simulink model "ecelp_sq"  (Simulink 6.1)
settings: Solver=FixedStepDiscrete  SolverMode=SingleTasking  StartTime=0.0  StopTime=3  RelTol=1e-3
PreLoadFcn:
  | load lpcvocoder.mat;
undefined symbols (not defined in the file): magnitude, poly2lsf
libraries: simulink x26, dspquant2 x26, dspindex x18, dspcelplib x14, dsparch4 x12, dspstat3 x10, dspsrcs4 x9, dspsigops x7, dsplp x5, dspmtrx3 x3, dspbuff3 x2, dspsolvers x1
(part 1 of 4)
settings Model: RequirementInfo=9  CovMetricSettings=d  Creator=The MathWorks Inc.  LastModifiedBy=igor  ExtModeTrigMode=oneshot  ExtModeArmWhenConnect=off  ExtModeAutoUpdateStatusClock=off  ProdHWDeviceType=Specified
settings DataIOCC: LimitDataPoints=off  SaveFormat=Structure  SaveOutput=off  SaveTime=off  SignalLoggingName=sigsOut
settings OptimizationCC: BlockReduction=off  BooleanDataType=off  InlineInvariantSignals=off
settings DebuggingCC: CheckExecutionContextPreStartOutputMsg=on  CheckExecutionContextRuntimeOutputMsg=on  InheritedTsInSrcMsg=none  IntegerOverflowMsg=none
settings HardwareCC: ProdHWDeviceType=Specified

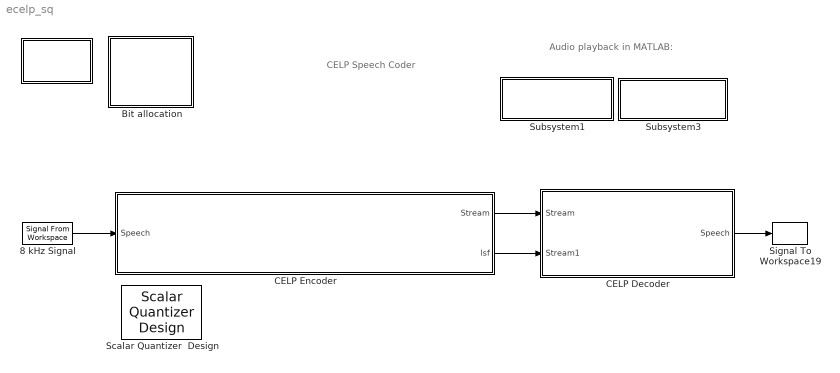
== system ecelp_sq ==
  note: CELP Speech Coder
  note: Audio playback in MATLAB:
  " " : Subsystem
      mask Type: CELP Coder Demo Info
      mask Display: disp('Info')
  "  Bit allocation" : Subsystem  mask(Bit Allocation){bitLSF1to3=10, bitLSF4to6=10, bitLSF7to10=10, bitD=7, bitBeta=6, bitSignGain=4, bitPhase=17, bitAlpha=6}
      mask prompts: bitLSF1to3 "Number of bits for 1st LSF subvector (1 to 3) (per frame):"; bitLSF4to6 "Number of bits for 2nd LSF subvector (4 to 6) (per frame):"; bitLSF7to10 "Number of bits for 3rd LSF subvector (7 to 10) (per frame):"; bitD "Number of bits for Pitch Delay, D (per subframe):"; bitBeta "Number of bits for Pitch Gain, Beta (per subframe):"; bitSignGain "Number of bits for sign of 4 FCB pulses (per subframe):"; bitPhase "Number of bits for position of 4 FCB pulses (per subframe):"; bitAlpha "Number of bits for FCB Gain, Alpha (per subframe):"
      mask help: Bit allocation for the speech coder designed for narrowband speech (sampling frequency 8 KHz) having a frame length of 160 samples and a subframe length of 40 samples (4 subframes per frame).
      mask StyleString: popup(10),popup(10),popup(10),popup(7),popup(6),popup(4),popup(17),popup(6)
      mask Display: disp('Bitrate\n9500 bps')
  8 kHz Signal : dspsrcs4/Signal From Workspace  X=Speech  Ts=1/8000  nsamps=160  OutputAfterFinalValue=Setting to zero
  CELP Decoder : Subsystem
      mask Display:
      | disp('   CELP\n     Decoder')
      | port_label( 'output',1,'Speech' )
      | port_label( 'input', 1, 'dLSFpfc' )
      | port_label( 'input',2,'Other stream' )
  CELP Encoder : Subsystem
      mask Display:
      | disp('CELP\nEncoder')
      | port_label('input',1,'Speech')
      | port_label('output',1,'dequa_LSF per frame content')
      | port_label('output',2,'Other stream')
  Scalar Quantizer  Design : dspquant2/Scalar Quantizer  Design
  Signal To Workspace19 : dspsnks4/Signal To Workspace  VariableName=y_lpc  FrameMode=Concatenate frames (2-D array)
      settings: FixptAsFi=off
  Subsystem1 : Subsystem
      settings: OpenFcn=if exist('Speech','var'), soundsc(Speech,8000); else errordlg('Data not found in workspace - reload demo model.','Signal Processing Blockset Demo Error'); end
      mask Display: disp('Original\nSignal')
  Subsystem3 : Subsystem
      settings: OpenFcn=if exist('y_lpc','var'), soundsc(y_lpc,8000); else uiwait(errordlg('You must run the simulation first.','Signal Processing Blockset Demo Error','modal')); end
      mask Display: disp('Processed\nSignal')
  wires:
  8 kHz Signal/1 -> CELP Encoder/1(Speech)
  CELP Decoder/1(Speech) -> Signal To Workspace19/1
  CELP Encoder/1(Stream) -> CELP Decoder/1(Stream)
  CELP Encoder/2(lsf) -> CELP Decoder/2(Stream1)

== system ecelp_sq/  ==
  note: Code Excited Linear Prediction (CELP) speech coder demo
      |
      | This demo contains a CELP coder composed of an encoder and a decoder.
      |
      | In the encoder, we estimate the parameters of the short-term synthesis
      | filter, the long-term pitch filter and the innovation signal.
      |
      | Using the linear prediction (LP) analysis followed by the quantization and
      | the interpolation of the LSF parameters we calculate the synthesis filter
      | coefficients for each subframe.
      |
      | By applying open loop pitch analysis on the LPC residual signal in each
      | subframe we estimate the pitch predictor delay and the pitch gain
      | parameters.
      |
      | By applying a search on the pitch predictor residual we specify the
      | location and the signs of the FCB (Fixed Code Book) pulses and the FCB
      | gain.
      |
      | To illustrate how the LPC and the pitch analyses remove the short-term and
      | long-term redundancies in the speech signal, the LPC and the pitch residual
      | signals are visualized.
      |
      | The decoder re-synthesizes the speech signal based on the CELP coder
      | parameters contained in the data stream.
      |
      | In this simulation, the speech signal is divided into frames of size 20 ms
      | (160 samples) and each frame is subdivided into four subframes of 5 ms (40
      | samples) each. The bit allocation for each parameter of the coder can be
      | found by double clicking on the 'Bit Allocation' block.
      |
      | The speech phrase used in this demo is from the Harvard list of
      | phonetically balanced sentences, list 14, phrase 8:
      | "Clothes and lodging are free to new men."

== system ecelp_sq/  Bit allocation ==

== system ecelp_sq/CELP Decoder ==
  Stream : Inport  Port=1  LatchInput=off
  Stream1 : Inport  Port=2  LatchInput=off
  Concatenation of subframes to form frame : simulink/Math Operations/Reshape  OutputDimensionality=Customize  OutputDimensions=[160,1]
  Decoding of Data-Stream : dspindex/Multiport Selector  rowsOrCols=Columns  idxCellArray={ 4-3:7-3,8-3:11-3,12-3:27-3,28-3:43-3,44-3:47-3 }  idxErrMode=Clip Index
  Frame to subframe : simulink/Math Operations/Reshape  OutputDimensionality=Customize  OutputDimensions=[4,4]
  LSF Interpolation : Subsystem
  LSF dequantization : Subsystem
  Reshape2 : simulink/Math Operations/Reshape  OutputDimensionality=Customize  OutputDimensions=[4,4]
  Subframe Synthesis : Subsystem  TreatAsAtomicUnit=on
  Speech : Outport
  wires:
  LSF Interpolation/1(LSFinterp) -> Subframe Synthesis/1(lSF_4CH)
  Subframe Synthesis/1(Sigout) -> Concatenation of subframes to form frame/1
  LSF dequantization/1(LSF) -> LSF Interpolation/1(LSF)
  Decoding of Data-Stream/3 -> Frame to subframe/1
  Decoding of Data-Stream/4 -> Reshape2/1
  Decoding of Data-Stream/5 -> Subframe Synthesis/6(Idx_FCBgain)
  Frame to subframe/1 -> Subframe Synthesis/4(4Position)
  Reshape2/1 -> Subframe Synthesis/5(4SignBit)
  Stream/1 -> Decoding of Data-Stream/1
  Concatenation of subframes to form frame/1 -> Speech/1
  Stream1/1 -> LSF dequantization/1(Idx_lsf1to3)
  Decoding of Data-Stream/1 -> Subframe Synthesis/2(Idx_D)
  Decoding of Data-Stream/2 -> Subframe Synthesis/3(Idx_beta)

== system ecelp_sq/CELP Encoder ==
  Speech : Inport  Port=1  LatchInput=off
  DC bias removal : dsparch4/Digital Filter  DialogController=dspDDGCreate  DialogControllerArgs=DataTag12  TypePopup=IIR (poles & zeros)  IIRFiltStruct=Direct form II transposed  AllPoleFiltStruct=Direct form  FIRFiltStruct=Direct form  CoeffSource=Specify via dialog  NumCoeffs="[ 0.9201   -1.8401    0.9201]"  DenCoeffs="[ 1.0000   -1.8337    0.8465]"  BiQuadCoeffs=[1 0.3 0.4 1 0.1 0.2]  LatticeCoeffs=[0.2 0.4]  denIgnore=on  FiltPerSampPopup=One filter per frame  IC=0  ICnum=0  ICden=0  roundingMode=Floor  overflowMode=off  ScaleValues=1  scaleValueFracLength=14  stageInFracLength=15  stageOutFracLength=15
  Data-Stream generation : simulink/Math Operations/Matrix Concatenation  numInports=5  catMethod=Horizontal
  Frame Analysis : Subsystem
  Subframe Analysis : Subsystem  TreatAsAtomicUnit=on
  Stream : Outport
  lsf : Outport  Port=2
  wires:
  Frame Analysis/2(LSF) -> Subframe Analysis/1(LSF)
  DC bias removal/1 -> Frame Analysis/1(FilteredSp), Subframe Analysis/2(Speech)
  Subframe Analysis/5(Idx_FCBgain) -> Data-Stream generation/5
  Data-Stream generation/1 -> Stream/1
  Speech/1 -> DC bias removal/1
  Subframe Analysis/1(Idx_D) -> Data-Stream generation/1
  Subframe Analysis/2(Idx_Beta) -> Data-Stream generation/2
  Subframe Analysis/3(4Position) -> Data-Stream generation/3
  Subframe Analysis/4(4SignBit) -> Data-Stream generation/4
  Frame Analysis/1(IdxLSF) -> lsf/1

== system ecelp_sq/Subsystem1 ==

== system ecelp_sq/Subsystem3 ==

== system ecelp_sq/CELP Decoder/LSF Interpolation ==
  note: LSF Interpolation
  LSF : Inport  Port=1  LatchInput=off
  Delay : dspsigops/Delay  Orientation=down  dly_unit=Frames  delay=1  ic_detail=on  dif_ic_for_ch=off  dif_ic_for_dly=on  ic=(poly2lsf([1 zeros(1,10)])).'  reset_popup=None
  Frame Status : FrameConversion
  Frame Status1 : FrameConversion  OutFrame=Sample based
  Gain : Gain  Orientation=down  Gain=1/4  SaturateOnIntegerOverflow=on
  Matrix Concatenation : simulink/Math Operations/Matrix Concatenation  numInports=4  catMethod=Horizontal
  Sum : Sum  Orientation=down  Inputs=|+-  SaturateOnIntegerOverflow=on
  Sum1 : Sum  Orientation=down  Inputs=++|  SaturateOnIntegerOverflow=on
  Sum2 : Sum  Orientation=down  Inputs=++|  SaturateOnIntegerOverflow=on
  Sum3 : Sum  Inputs=++|  SaturateOnIntegerOverflow=on
  LSFinterp : Outport
  wires:
  LSF/1 -> Frame Status/1
  Sum/1 -> Gain/1
  Sum1/1 -> Matrix Concatenation/1, Sum2/2
  Matrix Concatenation/1 -> Frame Status1/1
  Sum2/1 -> Sum3/1, Matrix Concatenation/2
  Sum3/1 -> Matrix Concatenation/3
  Delay/1 -> Sum1/2, Sum/2
  Gain/1 -> Sum1/1, Sum2/1, Sum3/2
  Frame Status/1 -> Sum/1, Delay/1, Matrix Concatenation/4
  Frame Status1/1 -> LSFinterp/1

== system ecelp_sq/CELP Decoder/LSF dequantization ==
  note: Decoding of LSF sub-vectors
  Idx_lsf1to3 : Inport  Port=1  LatchInput=off
  Sort : dspstat3/Sort  DialogController=dspDDGCreate  DialogControllerArgs=DataTag0  otype=Value  dir=Ascending  sortAlg=Quick sort  roundingMode=Floor  overflowMode=off
  LSF : Outport
  wires:
  Idx_lsf1to3/1 -> Sort/1
  Sort/1 -> LSF/1

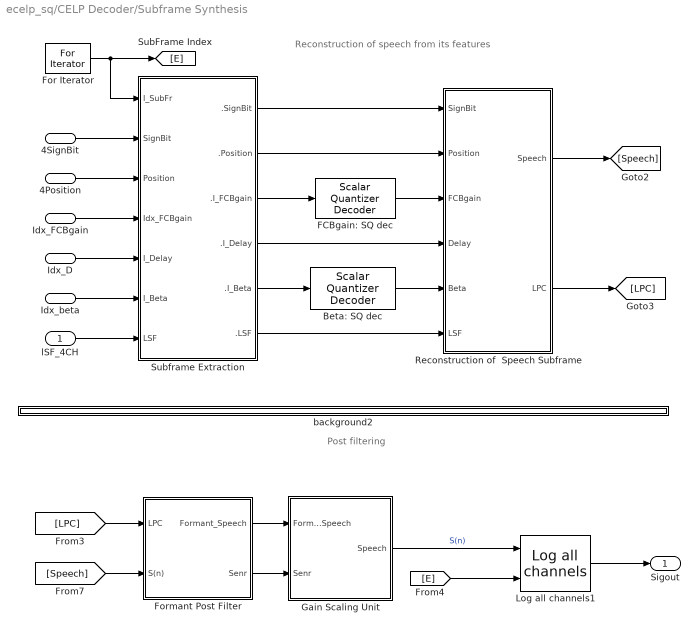
== system ecelp_sq/CELP Decoder/Subframe Synthesis ==
  note: Post filtering
  note: Reconstruction of speech from its features
  lSF_4CH : Inport  Port=1  LatchInput=off
  Idx_D : Inport  Port=2  LatchInput=off
  Idx_beta : Inport  Port=3  LatchInput=off
  4Position : Inport  Port=4  LatchInput=off
  4SignBit : Inport  Port=5  LatchInput=off
  Idx_FCBgain : Inport  Port=6  LatchInput=off
  Beta: SQ dec : dspquant2/Scalar Quantizer Decoder  CBsource=Specify via dialog  invalidin=Clip  codebook="[-1082.3569     -246.64044     -206.60177     -119.68735     -118.12987     -109.71395     -107.74187     -101.39102     -96.836918     -91.269156     -86.372177     -83.198634     -82.501047     -77.265358     -76.499561     -74.506154     -73.162943     -72.064354     -69.588398     -67.441995     -64.571558     -63.949501     -62.716478     -61.876738     -61.311021     -60.518343     -58.650854     -57.975792     -56.936942     -56.282238     -55.386427     -54.862852     -53.494072      -52.94422     -52.032961      -50.72662     -48.968103      -46.10807       -42.6265     -39.065568     -34.843913     -30.198965     -25.969732     -21.578415     -17.256677     -13.047571     -8.5748944     -4.8378646     -2.2872972    -0.86065481    -0.37978458     0.45579633     0.94262874      4.3421606      12.379451      23.629803       37.40066      54.817595      74.624825      93.641473      110.49643      136.97269      179.36351      233.98073]"  dataType=double  isSigned=on  wordLen=16  udDataType=sfix(16)  fracBitsMode=Best precision  numFracBits=11
  FCBgain: SQ dec : dspquant2/Scalar Quantizer Decoder  CBsource=Specify via dialog  invalidin=Clip  codebook="[-0.056021   -0.044097   -0.036312   -0.032845   -0.027656   -0.024334   -0.021157   -0.016236   -0.012644   -0.009939  -0.0075682   -0.005381    -0.00346  -0.0018555 -0.00067033  0.00028187   0.0011099   0.0020196   0.0029919   0.0040377   0.0051592   0.0063683   0.0076408   0.0090117    0.010466    0.012026     0.01376    0.015654    0.017725     0.01998    0.022452    0.025171    0.028043    0.031282    0.034713    0.038275    0.042246    0.046745    0.051613     0.05696     0.06287    0.069146    0.075778    0.082252     0.08972    0.096123     0.10068     0.10407     0.10799     0.11193     0.11573     0.11868     0.12213     0.12664     0.13004     0.13378     0.13772      0.1425     0.14445     0.14843     0.16231     0.16577      0.1698     0.18011]"  dataType=double  isSigned=on  wordLen=16  udDataType=sfix(16)  fracBitsMode=Best precision  numFracBits=11
  For Iterator : ForIterator  IterationLimit=4
  Formant Post Filter : Subsystem
  Gain Scaling Unit : Subsystem
  Log all channels1 : dspcelplib/Log all channels  outType=Matrix  numRow=40  numCol=4  dType=double
  Reconstruction of  Speech Subframe : Subsystem
  Subframe Extraction : Subsystem
  background2 : Subsystem
      mask Display: disp('')
  Sigout : Outport
  wires:
  For Iterator/1 -> [E], Subframe Extraction/1(I_SubFr)
  Subframe Extraction/6(.LSF) -> Reconstruction of  Speech Subframe/6(LSF)
  lSF_4CH/1 -> Subframe Extraction/7(LSF)
  Reconstruction of  Speech Subframe/1(Speech) -> [Speech]
  Idx_beta/1 -> Subframe Extraction/6(I_Beta)
  Subframe Extraction/5(.I_Beta) -> Beta: SQ dec/1
  Idx_D/1 -> Subframe Extraction/5(I_Delay)
  [Speech] -> Formant Post Filter/2(S(n))
  Formant Post Filter/2(Senr) -> Gain Scaling Unit/2(Senr)
  Formant Post Filter/1(Formant_Speech) -> Gain Scaling Unit/1(Formant_Speech)
  [LPC] -> Formant Post Filter/1(LPC)
  Gain Scaling Unit/1(Speech) -> Log all channels1/1  "S(n)"
  Log all channels1/1 -> Sigout/1
  [E] -> Log all channels1/2
  Subframe Extraction/2(.Position) -> Reconstruction of  Speech Subframe/2(Position)
  Subframe Extraction/1(.SignBit) -> Reconstruction of  Speech Subframe/1(SignBit)
  4Position/1 -> Subframe Extraction/3(Position)
  4SignBit/1 -> Subframe Extraction/2(SignBit)
  Idx_FCBgain/1 -> Subframe Extraction/4(Idx_FCBgain)
  Subframe Extraction/3(.I_FCBgain) -> FCBgain: SQ dec/1
  Reconstruction of  Speech Subframe/2(LPC) -> [LPC]
  FCBgain: SQ dec/1 -> Reconstruction of  Speech Subframe/3(FCBgain)
  Subframe Extraction/4(.I_Delay) -> Reconstruction of  Speech Subframe/4(Delay)
  Beta: SQ dec/1 -> Reconstruction of  Speech Subframe/5(Beta)

== system ecelp_sq/CELP Encoder/Frame Analysis ==
  FilteredSp : Inport  Port=1  LatchInput=off
  " " : Subsystem
      mask Type: CELP Coder Demo Info
      mask Display: disp('Info')
  Classical LPC analysis : Subsystem
      mask Display:
      | disp('LPC\nAnalysis');
      | port_label('input',1,'speech');
      | port_label('output',1,'LPC');
  LSF Interpolation : Subsystem
  LSF Vector Quantization : Subsystem
  IdxLSF : Outport
  LSF : Outport  Port=2
  wires:
  Classical LPC analysis/1(LPC) -> LSF Vector Quantization/1(LPC)
  LSF Vector Quantization/1(qLSF) -> LSF Interpolation/1(LSF)
  FilteredSp/1 -> Classical LPC analysis/1(Speech)
  LSF Interpolation/1(LSFinterp) -> LSF/1
  LSF Vector Quantization/2(IdxLSF) -> IdxLSF/1

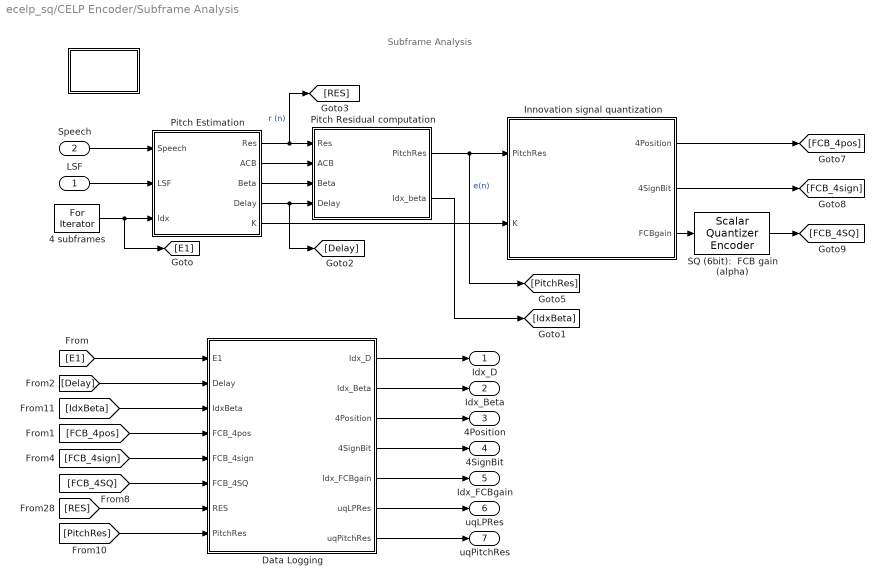
== system ecelp_sq/CELP Encoder/Subframe Analysis ==
  note: Subframe Analysis
  LSF : Inport  Port=1  LatchInput=off
  Speech : Inport  Port=2  LatchInput=off
  " " : Subsystem
      mask Type: CELP Coder Demo Info
      mask Display: disp('Info')
  4 subframes : ForIterator  IterationLimit=4
  Data Logging : Subsystem
  Innovation signal quantization : Subsystem
      mask Display:
      | disp('Pitch\nResidual\nQuantizer');
      | port_label('input',1,'PitchRes');
      | port_label('input',2,'K');
      | port_label('output',1,'4Position');
      | port_label('output',2,'4SignBit');
      | port_label('output',3,'FCBgain');
  Pitch Estimation : Subsystem
  Pitch Residual computation : Subsystem
  SQ (6bit):  FCB gain (alpha) : dspquant2/Scalar Quantizer Encoder  paramSrc=Specify via dialog  partType=Unbounded  BBoundary=[1:10]  UBoundary="[-0.050059   -0.040204   -0.034578   -0.030251   -0.025995   -0.022746   -0.018697    -0.01444   -0.011291  -0.0087536  -0.0064746  -0.0044205  -0.0026578  -0.0012629 -0.00019423  0.00069587   0.0015648   0.0025058   0.0035148   0.0045985   0.0057637   0.0070046   0.0083263   0.0097388    0.011246    0.012893    0.014707    0.016689    0.018853    0.021216    0.023812    0.026607    0.029663    0.032998    0.036494    0.040261    0.044496    0.049179    0.054286    0.059915    0.066008    0.072462    0.079015    0.085986    0.092922    0.098403     0.10238     0.10603     0.10996     0.11383      0.1172     0.12041     0.12439     0.12834     0.13191     0.13575     0.14011     0.14347     0.14644     0.15537     0.16404     0.16779     0.17495]"  SearchMethod=Binary  tieBreakRule=Choose the lower index  outQU=off  outQError=off  codebook="[-1082.3569     -246.64044     -206.60177     -119.68735     -118.12987     -109.71395     -107.74187     -101.39102     -96.836918     -91.269156     -86.372177     -83.198634     -82.501047     -77.265358     -76.499561     -74.506154     -73.162943     -72.064354     -69.588398     -67.441995     -64.571558     -63.949501     -62.716478     -61.876738     -61.311021     -60.518343     -58.650854     -57.975792     -56.936942     -56.282238     -55.386427     -54.862852     -53.494072      -52.94422     -52.032961      -50.72662     -48.968103      -46.10807       -42.6265     -39.065568     -34.843913     -30.198965     -25.969732     -21.578415     -17.256677     -13.047571     -8.5748944     -4.8378646     -2.2872972    -0.86065481    -0.37978458     0.45579633     0.94262874      4.3421606      12.379451      23.629803       37.40066      54.817595      74.624825      93.641473      110.49643      136.97269      179.36351      233.98073]"  outStatus=off  invalidin=Clip  idtype=int32  roundingMode=Floor  overflowMode=off
  Idx_D : Outport
  Idx_Beta : Outport  Port=2
  4Position : Outport  Port=3
  4SignBit : Outport  Port=4
  Idx_FCBgain : Outport  Port=5
  uqLPRes : Outport  Port=6
  uqPitchRes : Outport  Port=7
  wires:
  4 subframes/1 -> [E1], Pitch Estimation/3(Idx)
  Speech/1 -> Pitch Estimation/1(Speech)
  LSF/1 -> Pitch Estimation/2(LSF)
  Data Logging/1(Idx_D) -> Idx_D/1
  [Delay] -> Data Logging/2(Delay)
  Pitch Residual computation/1(PitchRes) -> [PitchRes], Innovation signal quantization/1(PitchRes)  "e(n)"
  Data Logging/2(Idx_Beta) -> Idx_Beta/1
  Data Logging/6(uqLPRes) -> uqLPRes/1
  Data Logging/7(uqPitchRes) -> uqPitchRes/1
  [PitchRes] -> Data Logging/8(PitchRes)
  [RES] -> Data Logging/7(RES)
  Pitch Estimation/5(K) -> Innovation signal quantization/2(K)
  Innovation signal quantization/3(FCBgain) -> SQ (6bit):  FCB gain (alpha)/1
  Data Logging/5(Idx_FCBgain) -> Idx_FCBgain/1
  Data Logging/3(4Position) -> 4Position/1
  Data Logging/4(4SignBit) -> 4SignBit/1
  Pitch Estimation/1(Res) -> Pitch Residual computation/1(Res), [RES]  "r (n)"
  Pitch Estimation/2(ACB) -> Pitch Residual computation/2(ACB)
  Pitch Estimation/3(Beta) -> Pitch Residual computation/3(Beta)
  Pitch Estimation/4(Delay) -> Pitch Residual computation/4(Delay), [Delay]
  Innovation signal quantization/1(4Position) -> [FCB_4pos]
  [FCB_4pos] -> Data Logging/4(FCB_4pos)
  Innovation signal quantization/2(4SignBit) -> [FCB_4sign]
  [FCB_4sign] -> Data Logging/5(FCB_4sign)
  SQ (6bit):  FCB gain (alpha)/1 -> [FCB_4SQ]
  [FCB_4SQ] -> Data Logging/6(FCB_4SQ)
  Pitch Residual computation/2(Idx_beta) -> [IdxBeta]
  [IdxBeta] -> Data Logging/3(IdxBeta)
  [E1] -> Data Logging/1(E1)

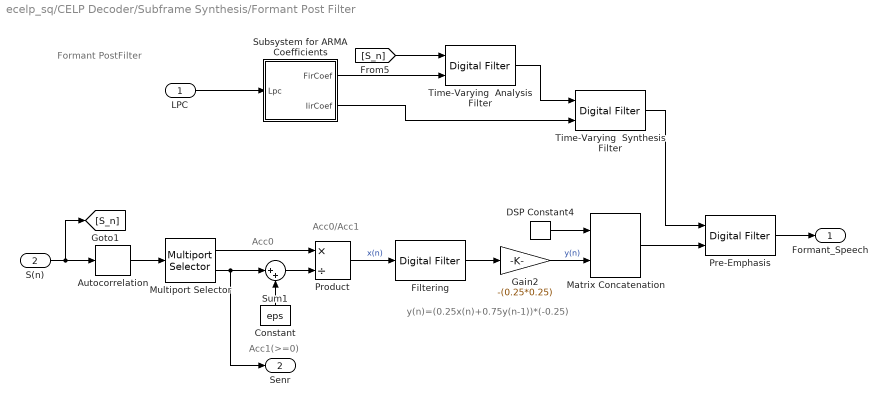
== system ecelp_sq/CELP Decoder/Subframe Synthesis/Formant Post Filter ==
  note: Formant PostFilter
  note: Acc0/Acc1
  note: Acc0
  note: Acc1(>=0)
  note: y(n)=(0.25x(n)+0.75y(n-1))*(-0.25)
  LPC : Inport  Port=1  LatchInput=off
  S(n) : Inport  Port=2  LatchInput=off
  Autocorrelation : dspstat3/Autocorrelation  DialogController=dspDDGCreate  DialogControllerArgs=DataTag1  AllPositiveLags=off  maxlag=1  bias=None  domain=Time  roundingMode=Floor  overflowMode=off
  Constant : Constant  Orientation=up  Value=eps
  DSP Constant4 : dspsrcs4/DSP Constant  Value=1  SampleMode=Discrete  discreteOutput=Sample-based  continuousOutput=Sample-based  sampTime=-1  framePeriod=-1  dataType=double  isSigned=on  wordLen=16  udDataType=sfix(16)  fracBitsMode=Best precision  numFracBits=15  InterpretAs1D=-inf  Ts=-inf  FramebasedOutput=-inf
      settings: additionalParams=on
  Filtering : dsparch4/Digital Filter  DialogController=dspDDGCreate  DialogControllerArgs=DataTag2  TypePopup=IIR (all poles)  IIRFiltStruct=Direct form II transposed  AllPoleFiltStruct=Direct form  FIRFiltStruct=Direct form  CoeffSource=Specify via dialog  NumCoeffs=[1 -.95]  DenCoeffs=[1 -0.75]  BiQuadCoeffs=[1 0.3 0.4 1 0.1 0.2]  LatticeCoeffs=[0.2 0.4]  denIgnore=on  FiltPerSampPopup=One filter per frame  IC=0  ICnum=0  ICden=0  roundingMode=Floor  overflowMode=off  ScaleValues=1  scaleValueFracLength=14  stageInFracLength=15  stageOutFracLength=15
  Gain2 : Gain  Gain=-(0.25*0.25)  SaturateOnIntegerOverflow=on
  Matrix Concatenation : simulink/Math Operations/Matrix Concatenation  numInports=2  catMethod=Vertical
  Multiport Selector : dspindex/Multiport Selector  rowsOrCols=Rows  idxCellArray={2,1}  idxErrMode=Clip Index
  Pre-Emphasis : dsparch4/Digital Filter  DialogController=dspDDGCreate  DialogControllerArgs=DataTag3  TypePopup=FIR (all zeros)  IIRFiltStruct=Direct form II transposed  AllPoleFiltStruct=Direct form  FIRFiltStruct=Direct form  CoeffSource=Input port(s)  NumCoeffs=[1 -.95]  DenCoeffs=[1 0.1]  BiQuadCoeffs=[1 0.3 0.4 1 0.1 0.2]  LatticeCoeffs=[0.2 0.4]  denIgnore=on  FiltPerSampPopup=One filter per frame  IC=0  ICnum=0  ICden=0  roundingMode=Floor  overflowMode=off  ScaleValues=1  scaleValueFracLength=14  stageInFracLength=15  stageOutFracLength=15
  Product : Product  Inputs=*/  SaturateOnIntegerOverflow=on  RndMeth=Zero  InputSameDT=on
  Subsystem for ARMA Coefficients : Subsystem
  Sum1 : Sum  Inputs=|++  SaturateOnIntegerOverflow=on  InputSameDT=on
  Time-Varying  Analysis Filter : dsparch4/Digital Filter  DialogController=dspDDGCreate  DialogControllerArgs=DataTag6  TypePopup=FIR (all zeros)  IIRFiltStruct=Direct form II transposed  AllPoleFiltStruct=Direct form  FIRFiltStruct=Direct form  CoeffSource=Input port(s)  NumCoeffs=[1 -.95]  DenCoeffs=[1 0.1]  BiQuadCoeffs=[1 0.3 0.4 1 0.1 0.2]  LatticeCoeffs=[0.2 0.4]  denIgnore=on  FiltPerSampPopup=One filter per frame  IC=0  ICnum=0  ICden=0  roundingMode=Floor  overflowMode=off  ScaleValues=1  scaleValueFracLength=14  stageInFracLength=15  stageOutFracLength=15
  Time-Varying  Synthesis Filter : dsparch4/Digital Filter  DialogController=dspDDGCreate  DialogControllerArgs=DataTag7  TypePopup=IIR (all poles)  IIRFiltStruct=Direct form II transposed  AllPoleFiltStruct=Direct form  FIRFiltStruct=Direct form  CoeffSource=Input port(s)  NumCoeffs=[1 -.95]  DenCoeffs=[1 0.1]  BiQuadCoeffs=[1 0.3 0.4 1 0.1 0.2]  LatticeCoeffs=[0.2 0.4]  denIgnore=on  FiltPerSampPopup=One filter per frame  IC=0  ICnum=0  ICden=0  roundingMode=Floor  overflowMode=off  ScaleValues=1  scaleValueFracLength=14  stageInFracLength=15  stageOutFracLength=15
  Formant_Speech : Outport
  Senr : Outport  Port=2
  wires:
  LPC/1 -> Subsystem for ARMA Coefficients/1(Lpc)
  Autocorrelation/1 -> Multiport Selector/1
  S(n)/1 -> Autocorrelation/1, [S_n]
  Subsystem for ARMA Coefficients/2(IirCoef) -> Time-Varying  Synthesis Filter/2
  Subsystem for ARMA Coefficients/1(FirCoef) -> Time-Varying  Analysis Filter/2
  Multiport Selector/2 -> Sum1/1, Senr/1
  Multiport Selector/1 -> Product/1
  Time-Varying  Analysis Filter/1 -> Time-Varying  Synthesis Filter/1
  [S_n] -> Time-Varying  Analysis Filter/1
  Time-Varying  Synthesis Filter/1 -> Pre-Emphasis/1
  Matrix Concatenation/1 -> Pre-Emphasis/2
  DSP Constant4/1 -> Matrix Concatenation/1
  Gain2/1 -> Matrix Concatenation/2  "y(n)"
  Pre-Emphasis/1 -> Formant_Speech/1
  Sum1/1 -> Product/2
  Constant/1 -> Sum1/2
  Product/1 -> Filtering/1  "x(n)"
  Filtering/1 -> Gain2/1

== system ecelp_sq/CELP Decoder/Subframe Synthesis/Gain Scaling Unit ==
  note: Gain Scaling Unit
  note: Senr
  note: Acc1
  Formant_Speech : Inport  Port=1  LatchInput=off
  Senr : Inport  Port=2  LatchInput=off
  0.0625 : dspsrcs4/DSP Constant  Value=1/16  SampleMode=Discrete  discreteOutput=Sample-based  continuousOutput=Sample-based  sampTime=-1  framePeriod=-1  dataType=Inherit from 'Constant value'  isSigned=on  wordLen=16  udDataType=sfix(16)  fracBitsMode=Best precision  numFracBits=15  InterpretAs1D=off  Ts=-1  FramebasedOutput=off
  1.0625 : Constant  Value=17/16
  Dot Product : simulink/Math Operations/Dot Product  OutDataType=sfix(16)  OutScaling=2^-10  DoSatur=on
  For Iterator Subsystem1 : Subsystem  TreatAsAtomicUnit=on
  Gain2 : Gain  Gain=1/16  SaturateOnIntegerOverflow=on
  Product : Product  Inputs=*/  SaturateOnIntegerOverflow=on  RndMeth=Zero  InputSameDT=on
  Product1 : Product  Inputs=3  SaturateOnIntegerOverflow=on  RndMeth=Zero  InputSameDT=on
  Switch1 : Switch  Threshold=1.175494351e-38  SaturateOnIntegerOverflow=on  InputSameDT=on
  sqrt(Senr/Acc1) : Math  Operator=sqrt  SaturateOnIntegerOverflow=on
  Speech : Outport
  wires:
  Senr/1 -> Product/1
  Switch1/1 -> For Iterator Subsystem1/1(ScalarGain)
  Gain2/1 -> Switch1/1
  0.0625/1 -> Switch1/3
  sqrt(Senr/Acc1)/1 -> Gain2/1
  Product/1 -> sqrt(Senr/Acc1)/1
  Dot Product/1 -> Switch1/2, Product/2
  Formant_Speech/1 -> Dot Product/1, Dot Product/2, Product1/2
  1.0625/1 -> Product1/3
  For Iterator Subsystem1/1(VectorGain) -> Product1/1
  Product1/1 -> Speech/1

== system ecelp_sq/CELP Decoder/Subframe Synthesis/Reconstruction of  Speech Subframe ==
  SignBit : Inport  Port=1  LatchInput=off
  Position : Inport  Port=2  LatchInput=off
  FCBgain : Inport  Port=3  LatchInput=off
  Delay : Inport  Port=4  LatchInput=off
  Beta : Inport  Port=5  LatchInput=off
  LSF : Inport  Port=6  LatchInput=off
  Harmonic Shaper : Subsystem
  LP Synthesis Filter : Subsystem
  Pitch synthesis : Subsystem
  Reconstruction of  Pitch Residual Signal : Subsystem
  Speech : Outport
  LPC : Outport  Port=2
  wires:
  Delay/1 -> Harmonic Shaper/2(Delay), Pitch synthesis/2(Delay)
  Beta/1 -> Harmonic Shaper/3(Beta), Pitch synthesis/3(Beta)
  Harmonic Shaper/1(OutRes) -> LP Synthesis Filter/1(Residual)
  Reconstruction of  Pitch Residual Signal/1(qPitchRes) -> Pitch synthesis/1(PitchRes)
  Pitch synthesis/1(LPRes) -> Harmonic Shaper/1(inRes)
  SignBit/1 -> Reconstruction of  Pitch Residual Signal/1(4SignBit)
  Position/1 -> Reconstruction of  Pitch Residual Signal/2(4Position)
  FCBgain/1 -> Reconstruction of  Pitch Residual Signal/3(FCBgain)
  LP Synthesis Filter/1(Sig) -> Speech/1  "S(n)"
  LSF/1 -> LP Synthesis Filter/2(LSF)
  LP Synthesis Filter/2(LPC) -> LPC/1

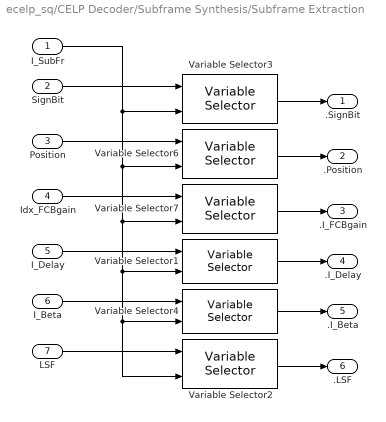
== system ecelp_sq/CELP Decoder/Subframe Synthesis/Subframe Extraction ==
  I_SubFr : Inport  Port=1  LatchInput=off
  SignBit : Inport  Port=2  LatchInput=off
  Position : Inport  Port=3  LatchInput=off
  Idx_FCBgain : Inport  Port=4  LatchInput=off
  I_Delay : Inport  Port=5  LatchInput=off
  I_Beta : Inport  Port=6  LatchInput=off
  LSF : Inport  Port=7  LatchInput=off
  Variable Selector1 : dspindex/Variable Selector  rowsOrCols=Columns  IdxMode=Variable  Elements=[1 3]  ZerOneIdxMode=One-based  errmode=Clip Index
  Variable Selector2 : dspindex/Variable Selector  rowsOrCols=Columns  IdxMode=Variable  Elements=[1 3]  ZerOneIdxMode=One-based  errmode=Clip Index
  Variable Selector3 : dspindex/Variable Selector  rowsOrCols=Columns  IdxMode=Variable  Elements=[1 3]  ZerOneIdxMode=One-based  errmode=Generate Error
  Variable Selector4 : dspindex/Variable Selector  rowsOrCols=Columns  IdxMode=Variable  Elements=[1 3]  ZerOneIdxMode=One-based  errmode=Clip Index
  Variable Selector6 : dspindex/Variable Selector  rowsOrCols=Columns  IdxMode=Variable  Elements=[1 3]  ZerOneIdxMode=One-based  errmode=Generate Error
  Variable Selector7 : dspindex/Variable Selector  rowsOrCols=Columns  IdxMode=Variable  Elements=[1 3]  ZerOneIdxMode=One-based  errmode=Generate Error
  .SignBit : Outport
  .Position : Outport  Port=2
  .I_FCBgain : Outport  Port=3
  .I_Delay : Outport  Port=4
  .I_Beta : Outport  Port=5
  .LSF : Outport  Port=6
  wires:
  I_SubFr/1 -> Variable Selector3/2, Variable Selector6/2, Variable Selector2/2, Variable Selector4/2, Variable Selector1/2, Variable Selector7/2
  SignBit/1 -> Variable Selector3/1
  Variable Selector3/1 -> .SignBit/1
  Position/1 -> Variable Selector6/1
  Variable Selector6/1 -> .Position/1
  Idx_FCBgain/1 -> Variable Selector7/1
  Variable Selector7/1 -> .I_FCBgain/1
  I_Delay/1 -> Variable Selector1/1
  Variable Selector1/1 -> .I_Delay/1
  I_Beta/1 -> Variable Selector4/1
  Variable Selector4/1 -> .I_Beta/1
  LSF/1 -> Variable Selector2/1
  Variable Selector2/1 -> .LSF/1

== system ecelp_sq/CELP Decoder/Subframe Synthesis/background2 ==

== system ecelp_sq/CELP Encoder/Frame Analysis/  ==
  note: Frame analysis is composed of three steps:
      |
      | 1. Classical LPC analysis
      | 2. Split vector quantization of LSF vector
      | 3. LSF interpolation

== system ecelp_sq/CELP Encoder/Frame Analysis/Classical LPC analysis ==
  note: LPC Analysis
  Speech : Inport  Port=1  LatchInput=off
  " " : Subsystem
      mask Type: CELP Coder Demo Info
      mask Display: disp('Info')
  Autocorrelation : dspstat3/Autocorrelation  DialogController=dspDDGCreate  DialogControllerArgs=DataTag13  AllPositiveLags=off  maxlag=10  bias=Biased  domain=Time  roundingMode=Floor  overflowMode=off
  Bandwidth Expansion : Subsystem  mask(Bandwidth Expansion){alpha=0.994}
      mask prompts: alpha "Bandwidth expansion factor:"
      mask help:
      | Generate autoregressive (AR) polynomial with bandwidth expanded relative to the bandwidth of the input AR polynomial.
      |
      | By reducing the radius of the roots in an autoregressive polynomial (i.e., scaling them towards the origin of the Z-plane), the bandwidth of the spectral peaks in the frequency response is expanded (flattened).  This operation is often referred to as "bandwidth expansion".
      |
      | Bandwidth expansion factor must be in the range [0,1], where 1.0 yields no changes to the roots of the polynomial.
      mask Help: web(dspbhelp);
      mask Display: fprintf('Bandwidth\nExpansion\n%g', alpha)
  Levinson- Durbin : dspsolvers/Levinson-Durbin  DialogController=dspDDGCreate  DialogControllerArgs=DataTag15  coeffOutFcn=A  outP=off  zeroInpHandling=on  firstCoeffMode=Binary point scaling  firstCoeffWordLength=16  firstCoeffFracLength=15  secondCoeffMode=Binary point scaling  secondCoeffWordLength=16  secondCoeffFracLength=15  roundingMode=Floor  overflowMode=off
      settings: allowOverrides=off
  Overlap Analysis Windows : dspbuff3/Buffer  N=240  V=80  ic=0
  Window : dspsigops/Window Function  DialogController=dspDDGCreate  DialogControllerArgs=DataTag16  winmode=Apply window to input  wintype=Hamming  sampmode=Continuous  samptime=1  N=64  Rs=50  beta=10  winsamp=Symmetric  UserWindow=hamming  OptParams=off  UserParams={1.0}  dataType=double  isSigned=on  wordLen=16  udDataType=sfix(16)  fracBitsMode=Best precision  numFracBits=15  roundingMode=Floor  overflowMode=off
  LPC : Outport
  wires:
  Overlap Analysis Windows/1 -> Window/1
  Autocorrelation/1 -> Levinson- Durbin/1
  Window/1 -> Autocorrelation/1
  Speech/1 -> Overlap Analysis Windows/1
  Levinson- Durbin/1 -> Bandwidth Expansion/1(In1)
  Bandwidth Expansion/1(Out1) -> LPC/1

== system ecelp_sq/CELP Encoder/Frame Analysis/LSF Interpolation ==
  note: LSF Interpolation
  LSF : Inport  Port=1  LatchInput=off
  " " : Subsystem
      mask Type: CELP Coder Demo Info
      mask Display: disp('Info')
  Delay : dspsigops/Delay  Orientation=down  dly_unit=Frames  delay=1  ic_detail=on  dif_ic_for_ch=off  dif_ic_for_dly=on  ic=(poly2lsf([1 zeros(1,10)])).'  reset_popup=None
  Frame Status : FrameConversion
  Frame Status1 : FrameConversion  OutFrame=Sample based
  Gain : Gain  Orientation=down  Gain=1/4  SaturateOnIntegerOverflow=on
  Matrix Concatenation : simulink/Math Operations/Matrix Concatenation  numInports=4  catMethod=Horizontal
  Sum : Sum  Orientation=down  Inputs=|+-  SaturateOnIntegerOverflow=on
  Sum1 : Sum  Orientation=down  Inputs=++|  SaturateOnIntegerOverflow=on
  Sum2 : Sum  Orientation=down  Inputs=++|  SaturateOnIntegerOverflow=on
  Sum3 : Sum  Inputs=++|  SaturateOnIntegerOverflow=on
  LSFinterp : Outport
  wires:
  Frame Status/1 -> Sum/1, Delay/1, Matrix Concatenation/4
  Sum/1 -> Gain/1
  Sum1/1 -> Matrix Concatenation/1, Sum2/2
  Matrix Concatenation/1 -> Frame Status1/1
  Sum2/1 -> Sum3/1, Matrix Concatenation/2
  Sum3/1 -> Matrix Concatenation/3
  Delay/1 -> Sum1/2, Sum/2
  Gain/1 -> Sum1/1, Sum2/1, Sum3/2
  LSF/1 -> Frame Status/1
  Frame Status1/1 -> LSFinterp/1

== system ecelp_sq/CELP Encoder/Frame Analysis/LSF Vector Quantization ==
  note: Split Vector Quantization of LSF vector
  LPC : Inport  Port=1  LatchInput=off
  " " : Subsystem
      mask Type: CELP Coder Demo Info
      mask Display: disp('Info')
  LPC to LSF  conversion : dsplp/LPC to LSF//LSP Conversion  output=LSF in range (0 pi)  NSteps=64  NBisects=4  RootStatus=off  correction=off  lastLSP=off  error=Ignore
  LSF xQ. : Subsystem
  Paliwal Weight  Computation : Subsystem
  Reshape1 : simulink/Math Operations/Reshape  OutputDimensionality=Column vector  OutputDimensions=[1,1]
  qLSF : Outport
  IdxLSF : Outport  Port=2
  wires:
  LPC/1 -> Reshape1/1
  Paliwal Weight  Computation/1(Weights) -> LSF xQ./2(W1to10)
  Reshape1/1 -> LPC to LSF  conversion/1, Paliwal Weight  Computation/2(LPC)
  LPC to LSF  conversion/1 -> Paliwal Weight  Computation/1(LSF), LSF xQ./1(U1to10)
  LSF xQ./1(qLSF) -> qLSF/1
  LSF xQ./2(IdxLSF) -> IdxLSF/1

== system ecelp_sq/CELP Encoder/Subframe Analysis/  ==
  note: Subframe analysis is composed of three steps:
      |
      | 1. Pitch estimation
      | 2. Pitch residual (innovation signal) computation
      | 3. Innovation signal quantization using fixed codebook

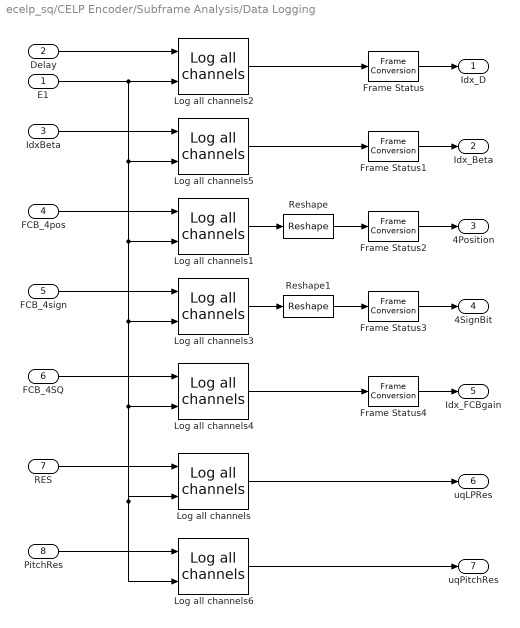
== system ecelp_sq/CELP Encoder/Subframe Analysis/Data Logging ==
  E1 : Inport  Port=1  LatchInput=off
  Delay : Inport  Port=2  LatchInput=off
  IdxBeta : Inport  Port=3  LatchInput=off
  FCB_4pos : Inport  Port=4  LatchInput=off
  FCB_4sign : Inport  Port=5  LatchInput=off
  FCB_4SQ : Inport  Port=6  LatchInput=off
  RES : Inport  Port=7  LatchInput=off
  PitchRes : Inport  Port=8  LatchInput=off
  Frame Status{,1..4} (5 alike) : FrameConversion  OutFrame=Sample based
  Log all channels : dspcelplib/Log all channels  outType=Matrix  numRow=40  numCol=4  dType=double
  Log all channels1 : dspcelplib/Log all channels  outType=Matrix  numRow=4  numCol=4  dType=int32
  Log all channels2 : dspcelplib/Log all channels  outType=Row vector  numRow=40  numCol=4  dType=int32
  Log all channels3 : dspcelplib/Log all channels  outType=Matrix  numRow=4  numCol=4  dType=int32
  Log all channels4 : dspcelplib/Log all channels  outType=Row vector  numRow=40  numCol=4  dType=int32
  Log all channels5 : dspcelplib/Log all channels  outType=Row vector  numRow=40  numCol=4  dType=int32
  Log all channels6 : dspcelplib/Log all channels  outType=Matrix  numRow=40  numCol=4  dType=double
  Reshape : simulink/Math Operations/Reshape  OutputDimensionality=Customize  OutputDimensions=[1,16]
  Reshape1 : simulink/Math Operations/Reshape  OutputDimensionality=Customize  OutputDimensions=[1,16]
  Idx_D : Outport
  Idx_Beta : Outport  Port=2
  4Position : Outport  Port=3
  4SignBit : Outport  Port=4
  Idx_FCBgain : Outport  Port=5
  uqLPRes : Outport  Port=6
  uqPitchRes : Outport  Port=7
  wires:
  E1/1 -> Log all channels/2, Log all channels6/2, Log all channels4/2, Log all channels3/2, Log all channels1/2, Log all channels5/2, Log all channels2/2
  Log all channels1/1 -> Reshape/1
  Log all channels3/1 -> Reshape1/1
  Delay/1 -> Log all channels2/1
  Log all channels2/1 -> Frame Status/1
  IdxBeta/1 -> Log all channels5/1
  Log all channels5/1 -> Frame Status1/1
  FCB_4pos/1 -> Log all channels1/1
  Reshape/1 -> Frame Status2/1
  FCB_4sign/1 -> Log all channels3/1
  Reshape1/1 -> Frame Status3/1
  FCB_4SQ/1 -> Log all channels4/1
  Log all channels4/1 -> Frame Status4/1
  RES/1 -> Log all channels/1
  Log all channels/1 -> uqLPRes/1
  PitchRes/1 -> Log all channels6/1
  Log all channels6/1 -> uqPitchRes/1
  Frame Status/1 -> Idx_D/1
  Frame Status1/1 -> Idx_Beta/1
  Frame Status2/1 -> 4Position/1
  Frame Status3/1 -> 4SignBit/1
  Frame Status4/1 -> Idx_FCBgain/1

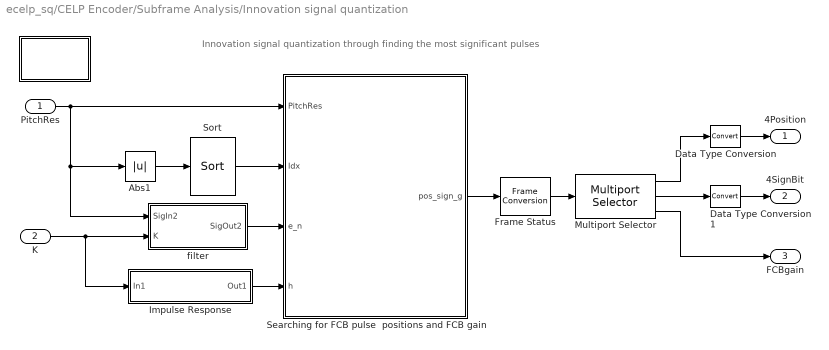
== system ecelp_sq/CELP Encoder/Subframe Analysis/Innovation signal quantization ==
  note: Innovation signal quantization through finding the most significant pulses
  PitchRes : Inport  Port=1  LatchInput=off
  K : Inport  Port=2  LatchInput=off
  " " : Subsystem
      mask Type: CELP Coder Demo Info
      mask Display: disp('Info')
  Abs1 : Abs  SaturateOnIntegerOverflow=on
  Data Type Conversion : DataTypeConversion  OutDataTypeMode=int32  SaturateOnIntegerOverflow=on  RndMeth=Zero
  Data Type Conversion1 : DataTypeConversion  OutDataTypeMode=int32  SaturateOnIntegerOverflow=on  RndMeth=Zero
  Frame Status : FrameConversion  OutFrame=Sample based
  Impulse Response : Subsystem
      mask Display:
      | disp('Impulse Response');
      | port_label('input',1,'K');
      | port_label('output',1,'h');
  Multiport Selector : dspindex/Multiport Selector  rowsOrCols=Rows  idxCellArray={ 1:4,5:8,9 }  idxErrMode=Generate Error
  Searching for FCB pulse  positions and FCB gain : Subsystem  TreatAsAtomicUnit=on
  Sort : dspstat3/Sort  DialogController=dspDDGCreate  DialogControllerArgs=DataTag21  otype=Index  dir=Descending  sortAlg=Quick sort  roundingMode=Floor  overflowMode=off
  filter : Subsystem  TreatAsAtomicUnit=on
      mask Display:
      | disp('Zero State\nIIR Lattice\nFilter');
      | port_label('input',1,'In');
      | port_label('input',2,'K');
      | port_label('output',1,'Out');
  4Position : Outport
  4SignBit : Outport  Port=2
  FCBgain : Outport  Port=3
  wires:
  Impulse Response/1(Out1) -> Searching for FCB pulse  positions and FCB gain/4(h)
  filter/1(SigOut2) -> Searching for FCB pulse  positions and FCB gain/3(e_n)
  K/1 -> Impulse Response/1(In1), filter/2(K)
  Multiport Selector/3 -> FCBgain/1
  Data Type Conversion1/1 -> 4SignBit/1
  Data Type Conversion/1 -> 4Position/1
  Sort/1 -> Searching for FCB pulse  positions and FCB gain/2(Idx)
  Abs1/1 -> Sort/1
  PitchRes/1 -> filter/1(SigIn2), Abs1/1, Searching for FCB pulse  positions and FCB gain/1(PitchRes)
  Multiport Selector/2 -> Data Type Conversion1/1
  Multiport Selector/1 -> Data Type Conversion/1
  Searching for FCB pulse  positions and FCB gain/1(pos_sign_g) -> Frame Status/1
  Frame Status/1 -> Multiport Selector/1

== system ecelp_sq/CELP Encoder/Subframe Analysis/Pitch Estimation ==
  note: Pitch Estimation
  Speech : Inport  Port=1  LatchInput=off
  LSF : Inport  Port=2  LatchInput=off
  Idx : Inport  Port=3  LatchInput=off
  " " : Subsystem
      mask Type: CELP Coder Demo Info
      mask Display: disp('Info')
  Frame Status : FrameConversion  OutFrame=Sample based
  LPC Residual Buffer : dspbuff3/Buffer  N=128+40+20-1  V=187-40  ic=0
  LPC Residual Calculation : Subsystem
  Open loop  Pitch estimation : Subsystem
  Subframe Extraction : Subsystem
  Res : Outport
  ACB : Outport  Port=2
  Beta : Outport  Port=3
  Delay : Outport  Port=4
  K : Outport  Port=5
  wires:
  Subframe Extraction/1(Speech.) -> LPC Residual Calculation/1(Speech)
  Subframe Extraction/2(LSF.) -> LPC Residual Calculation/2(LSF)
  LPC Residual Calculation/1(Residual) -> LPC Residual Buffer/1, Open loop  Pitch estimation/2(Res), Res/1  "r (n)"
  LPC Residual Buffer/1 -> Frame Status/1
  Speech/1 -> Subframe Extraction/1(Speech)
  Open loop  Pitch estimation/1(Beta) -> Beta/1
  LSF/1 -> Subframe Extraction/2(LSF)
  LPC Residual Calculation/2(K) -> K/1
  Idx/1 -> Subframe Extraction/3(SubFrIdx)
  Open loop  Pitch estimation/2(Delay) -> Delay/1
  Frame Status/1 -> ACB/1, Open loop  Pitch estimation/1(ACB)

== system ecelp_sq/CELP Encoder/Subframe Analysis/Pitch Residual computation ==
  note: r (n-D)
  note: beta.r (n-D)
  Res : Inport  Port=1  LatchInput=off
  ACB : Inport  Port=2  LatchInput=off
  Beta : Inport  Port=3  LatchInput=off
  Delay : Inport  Port=4  LatchInput=off
  " " : Subsystem
      mask Type: CELP Coder Demo Info
      mask Display: disp('Info')
  Adaptive codebook (ACB) vector candidate  generation : dspcelplib/Select Rows  numRows=40
  Frame Status : FrameConversion  OutFrame=Sample based
  Product : Product  SaturateOnIntegerOverflow=on  InputSameDT=on
  SQ (6bits):  Pitch gain (beta) : dspquant2/Scalar Quantizer Encoder  paramSrc=Specify via dialog  partType=Unbounded  BBoundary=[1:10]  UBoundary="[-664.4987     -226.6211     -163.1446     -118.9086     -113.9219     -108.7279     -104.5664     -99.11397     -94.05304     -88.82067     -84.78541     -82.84984      -79.8832     -76.88246     -75.50286     -73.83455     -72.61365     -70.82638      -68.5152     -66.00678     -64.26053     -63.33299     -62.29661     -61.59388     -60.91468      -59.5846     -58.31332     -57.45637     -56.60959     -55.83433     -55.12464     -54.17846     -53.21915     -52.48859     -51.37979     -49.84736     -47.53809     -44.36728     -40.84603     -36.95474     -32.52144     -28.08435     -23.77407     -19.41755     -15.15212     -10.81123      -6.70638     -3.562581     -1.573976    -0.6202197    0.03800587     0.6992125      2.642395      8.360806      18.00463      30.51523      46.10913      64.72121      84.13315       102.069      123.7346      158.1681      206.6721]"  SearchMethod=Binary  tieBreakRule=Choose the lower index  outQU=on  outQError=off  codebook="[-1082.3569     -246.64044     -206.60177     -119.68735     -118.12987     -109.71395     -107.74187     -101.39102     -96.836918     -91.269156     -86.372177     -83.198634     -82.501047     -77.265358     -76.499561     -74.506154     -73.162943     -72.064354     -69.588398     -67.441995     -64.571558     -63.949501     -62.716478     -61.876738     -61.311021     -60.518343     -58.650854     -57.975792     -56.936942     -56.282238     -55.386427     -54.862852     -53.494072      -52.94422     -52.032961      -50.72662     -48.968103      -46.10807       -42.6265     -39.065568     -34.843913     -30.198965     -25.969732     -21.578415     -17.256677     -13.047571     -8.5748944     -4.8378646     -2.2872972    -0.86065481    -0.37978458     0.45579633     0.94262874      4.3421606      12.379451      23.629803       37.40066      54.817595      74.624825      93.641473      110.49643      136.97269      179.36351      233.98073]"  outStatus=off  invalidin=Clip  idtype=int32  roundingMode=Floor  overflowMode=off
  Sum2 : Sum  Inputs=|+-  SaturateOnIntegerOverflow=on
  PitchRes : Outport
  Idx_beta : Outport  Port=2
  wires:
  ACB/1 -> Adaptive codebook (ACB) vector candidate  generation/1
  Sum2/1 -> Frame Status/1
  Res/1 -> Sum2/1  "r(n)"
  Delay/1 -> Adaptive codebook (ACB) vector candidate  generation/2
  Product/1 -> Sum2/2
  Adaptive codebook (ACB) vector candidate  generation/1 -> Product/1
  Beta/1 -> SQ (6bits):  Pitch gain (beta)/1
  SQ (6bits):  Pitch gain (beta)/2 -> Product/2
  SQ (6bits):  Pitch gain (beta)/1 -> Idx_beta/1
  Frame Status/1 -> PitchRes/1

== system ecelp_sq/CELP Decoder/Subframe Synthesis/Formant Post Filter/Subsystem for ARMA Coefficients ==
  Lpc : Inport  Port=1  LatchInput=off
  Bandwidth Expansion : Subsystem  mask(Bandwidth Expansion){alpha=0.65}
      mask prompts: alpha "Bandwidth expansion factor:"
      mask help:
      | Generate autoregressive (AR) polynomial with bandwidth expanded relative to the bandwidth of the input AR polynomial.
      |
      | By reducing the radius of the roots in an autoregressive polynomial (i.e., scaling them towards the origin of the Z-plane), the bandwidth of the spectral peaks in the frequency response is expanded (flattened).  This operation is often referred to as "bandwidth expansion".
      |
      | Bandwidth expansion factor must be in the range [0,1], where 1.0 yields no changes to the roots of the polynomial.
      mask Help: web(dspbhelp);
      mask Display: fprintf('Bandwidth\nExpansion\n%g', alpha)
  Bandwidth Expansion1 : Subsystem  mask(Bandwidth Expansion){alpha=0.75}
      mask prompts: alpha "Bandwidth expansion factor:"
      mask help:
      | Generate autoregressive (AR) polynomial with bandwidth expanded relative to the bandwidth of the input AR polynomial.
      |
      | By reducing the radius of the roots in an autoregressive polynomial (i.e., scaling them towards the origin of the Z-plane), the bandwidth of the spectral peaks in the frequency response is expanded (flattened).  This operation is often referred to as "bandwidth expansion".
      |
      | Bandwidth expansion factor must be in the range [0,1], where 1.0 yields no changes to the roots of the polynomial.
      mask Help: web(dspbhelp);
      mask Display: fprintf('Bandwidth\nExpansion\n%g', alpha)
  FirCoef : Outport
  IirCoef : Outport  Port=2
  wires:
  Lpc/1 -> Bandwidth Expansion/1(In1), Bandwidth Expansion1/1(In1)
  Bandwidth Expansion1/1(Out1) -> IirCoef/1
  Bandwidth Expansion/1(Out1) -> FirCoef/1

== system ecelp_sq/CELP Decoder/Subframe Synthesis/Gain Scaling Unit/For Iterator Subsystem1 ==
  note: g(n)
  note: y(n)
  note: y(n)=g(n)+0.9375y(n-1)
      | with IC=1
  note: Computation of gain scaling factor for each sample of the subframe
  ScalarGain : Inport  Port=1  LatchInput=off
  Assignment : Assignment  ElementSrc=External  Rows=-1  ColumnSrc=External
  Constant1 : Constant  Orientation=down  Value=zeros(40,1)  VectorParams1D=off
  For Iterator : ForIterator  IterationLimit=40
  filter : dsparch4/Digital Filter  DialogController=dspDDGCreate  DialogControllerArgs=DataTag8  TypePopup=IIR (all poles)  IIRFiltStruct=Direct form II transposed  AllPoleFiltStruct=Direct form  FIRFiltStruct=Direct form  CoeffSource=Specify via dialog  NumCoeffs=[1 -.95]  DenCoeffs="[1   -0.9375]"  BiQuadCoeffs=[1 0.3 0.4 1 0.1 0.2]  LatticeCoeffs=[0.2 0.4]  denIgnore=on  FiltPerSampPopup=One filter per frame  IC=1  ICnum=0  ICden=0  roundingMode=Floor  overflowMode=off  ScaleValues=1  scaleValueFracLength=14  stageInFracLength=15  stageOutFracLength=15
  VectorGain : Outport
  wires:
  For Iterator/1 -> Assignment/3
  Assignment/1 -> VectorGain/1
  Constant1/1 -> Assignment/1
  ScalarGain/1 -> filter/1
  filter/1 -> Assignment/2

== system ecelp_sq/CELP Decoder/Subframe Synthesis/Reconstruction of  Speech Subframe/Harmonic Shaper ==
  inRes : Inport  Port=1  LatchInput=off
  Delay : Inport  Port=2  LatchInput=off
  Beta : Inport  Port=3  LatchInput=off
  1-bz^(-D)2 : Subsystem  TreatAsAtomicUnit=on
  Energy normalization : Subsystem
  Pitch Synthesis Filtering 1/(1-b.z^(-D))2 : dsparch4/Digital Filter  DialogController=dspDDGCreate  DialogControllerArgs=DataTag9  TypePopup=IIR (all poles)  IIRFiltStruct=Direct form II transposed  AllPoleFiltStruct=Direct form  FIRFiltStruct=Direct form  CoeffSource=Input port(s)  NumCoeffs=[1 -.95]  DenCoeffs=[1 0.1]  BiQuadCoeffs=[1 0.3 0.4 1 0.1 0.2]  LatticeCoeffs=[0.2 0.4]  denIgnore=on  FiltPerSampPopup=One filter per frame  IC=0  ICnum=0  ICden=0  roundingMode=Floor  overflowMode=off  ScaleValues=1  scaleValueFracLength=14  stageInFracLength=15  stageOutFracLength=15
  OutRes : Outport
  wires:
  Pitch Synthesis Filtering 1/(1-b.z^(-D))2/1 -> Energy normalization/2(SigNew)
  inRes/1 -> Energy normalization/1(SigOrg), Pitch Synthesis Filtering 1/(1-b.z^(-D))2/1
  1-bz^(-D)2/1(Polynom) -> Pitch Synthesis Filtering 1/(1-b.z^(-D))2/2
  Delay/1 -> 1-bz^(-D)2/1(D_buf_1based)
  Beta/1 -> 1-bz^(-D)2/2(beta)
  Energy normalization/1(SigNew2) -> OutRes/1  "res"

== system ecelp_sq/CELP Decoder/Subframe Synthesis/Reconstruction of  Speech Subframe/LP Synthesis Filter ==
  Residual : Inport  Port=1  LatchInput=off
  LSF : Inport  Port=2  LatchInput=off
  LPC to/from RC : dsplp/LPC to//from RC  conversion=LPC to RC  perr=off  stability=off  error=Replace it with 1
  LSF/LSP to LPC Conversion : dsplp/LSF//LSP to LPC Conversion  input=LSF in range (0 pi)
  Time-Varying  Synthesis Filter 1/A(z) : dsparch4/Digital Filter  DialogController=dspDDGCreate  DialogControllerArgs=DataTag10  TypePopup=IIR (all poles)  IIRFiltStruct=Direct form II transposed  AllPoleFiltStruct=Lattice AR  FIRFiltStruct=Direct form  CoeffSource=Input port(s)  NumCoeffs=[1 -.95]  DenCoeffs=[1 0.1]  BiQuadCoeffs=[1 0.3 0.4 1 0.1 0.2]  LatticeCoeffs=[0.2 0.4]  denIgnore=off  FiltPerSampPopup=One filter per frame  IC=0  ICnum=0  ICden=0  roundingMode=Floor  overflowMode=off  ScaleValues=1  scaleValueFracLength=14  stageInFracLength=15  stageOutFracLength=15
  Sig : Outport
  LPC : Outport  Port=2
  wires:
  LSF/LSP to LPC Conversion/1 -> LPC to/from RC/1, LPC/1
  LPC to/from RC/1 -> Time-Varying  Synthesis Filter 1/A(z)/2
  Residual/1 -> Time-Varying  Synthesis Filter 1/A(z)/1
  Time-Varying  Synthesis Filter 1/A(z)/1 -> Sig/1  "S(n)"
  LSF/1 -> LSF/LSP to LPC Conversion/1
